simulink model "Streaming_LUT"  (R2024a)
settings: Solver=ode1  StartTime=0.0  StopTime=10  FixedStep=0.001  RelTol=1e-3  EnableMultiTasking=on
PreLoadFcn:
  | a = reshape(1:2800, [4 5 20 7]);
undefined symbols (not defined in the file): xi, yi, ZI
libraries: simulink x2
settings Model: Creator=The MathWorks, Inc.  LastModifiedBy=jjansev
settings SolverCC: AlgebraicLoopSolver=TrustRegion
settings DataIOCC: LimitDataPoints=on  SaveFormat=Array
settings OptimizationCC: ExpressionDepthLimit=2147483647  LifeSpan=inf
settings DebuggingCC: UnderspecifiedInitializationDetection=Classic  MergeDetectMultiDrivingBlocksExec=none  SolverPrmCheckMsg=warning  FcnCallInpInsideContextMsg=warning  UnconnectedInputMsg=warning  UnconnectedOutputMsg=warning  UnconnectedLineMsg=warning  StateNameClashWarn=warning  PregeneratedLibrarySubsystemCodeDiagnostic=none  SFUnexpectedBacktrackingDiag=warning  SFNoUnconditionalDefaultTransitionDiag=warning  SFExecutionAtInitializationDiag=none  ArithmeticOperatorsInVariantConditions=warning
settings HardwareCC: ProdBitPerPointer=32  ProdBitPerSizeT=32  ProdBitPerPtrDiffT=32  ProdLargestAtomicFloat=None  ProdIntDivRoundTo=Undefined  ProdEndianess=Unspecified  ProdWordSize=32  ProdHWDeviceType=32-bit Generic
settings ModelReferenceCC: EnableRefExpFcnMdlSchedulingChecks=on  PropagateSignalLabelsOutOfModel=off
settings SFSimCC: SimUseLocalCustomCode=off  CustomCodeUndefinedFunction=UseInterfaceOnly
settings RTWCC: RTWUseLocalCustomCode=off  GPUComputeCapability=3.5
settings CodeAppCC: StateflowObjectComments=on
settings GRTTargetCC: TargetLangStandard=C89/C90 (ANSI)  CombineOutputUpdateFcns=off  GRTInterface=on
settings ConfigComp: CovMetricSettings=dw  CovSaveCumulativeToWorkspaceVar=on  CovSaveSingleToWorkspaceVar=on  CovExternalEMLEnable=off

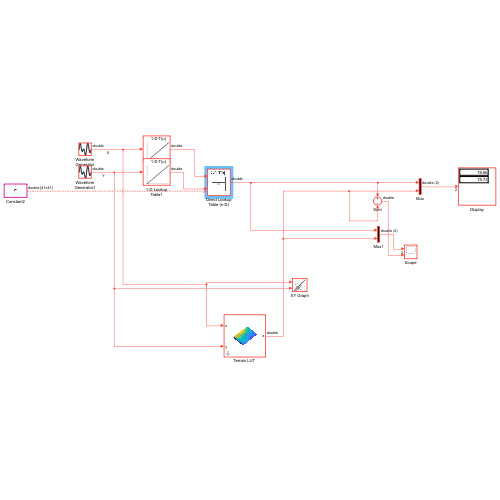
[thumbnail: Simulink's stored preview of the top-level diagram]
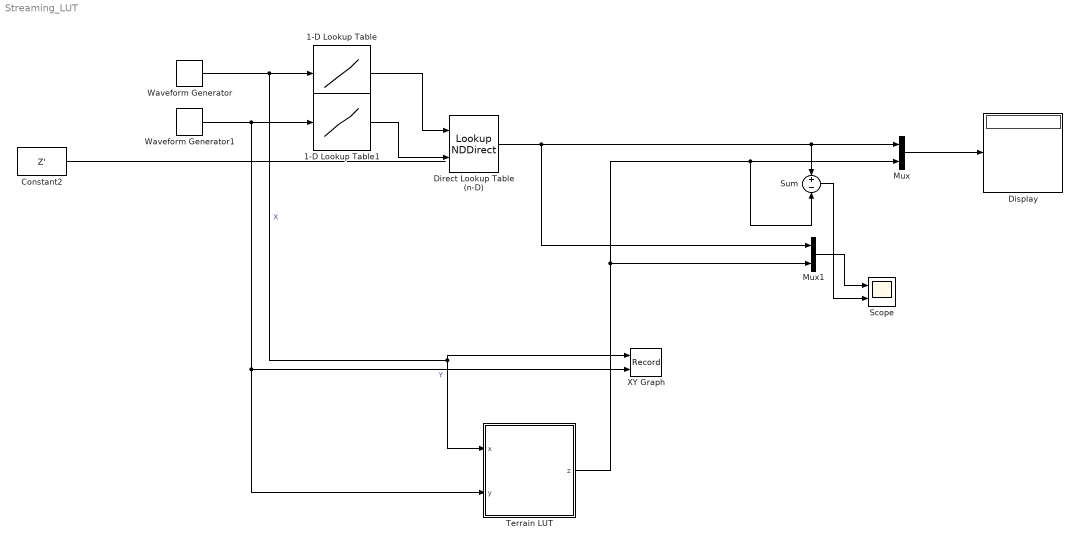
== system Streaming_LUT ==
  1-D Lookup Table : Lookup_n-D  NumberOfTableDimensions=1  BreakpointsForDimension1=[-10 10]  Table=[1 41]  InternalRulePriority=Speed  RndMeth=Simplest
  1-D Lookup Table1 : Lookup_n-D  NumberOfTableDimensions=1  BreakpointsForDimension1=[-10 10]  Table=[1 41]  InternalRulePriority=Speed  RndMeth=Simplest
  Constant2 : Constant  Value=Z'
  Direct Lookup Table (n-D) : LookupNDDirect  Table=Z'
  Display : Display
  Mux : Mux  Inputs=2
  Mux1 : Mux  Inputs=2
  Scope : Scope  NumInputPorts=2
  Sum : Sum  Inputs=+-
  "Terrain LUT " : Subsystem  AncestorBlock=|  mask{stlFileName='MRC_t.stl', resolution=5, color=[0.5 0.5 0.6], x_query=0, y_query=0, Int_method=Linear}
      | PC_GS_SSMB/TerrainFromSTL 
      | (Visuzalize GridSurface)
      mask prompts: stlFileName "STL Filename"; resolution "Resolution of the Grid surface [m]"; color "Color of the Grid-surface"; x_query "Position on x-axis to be polled for z-height (Frame F1)"; y_query "Position on y-axis to be polled for z-height (Frame F1)"; Int_method "Interpolation method Used of the Surface"
      mask init:
      | % Use set_param to set the parameter
      | [imageMatrix, xi, yi, ZI, Res_orig, z_query] = GenerateTerrainFromSTL(stlFileName, resolution, x_query, y_query, Int_method);
      mask Display: image(imageMatrix);
  Waveform Generator : simulink/Sources/Waveform Generator  OutMin=[]  OutMax=[]  OutDataTypeStr=double  SelectedSignal=1  Signals=sin(10.0,5,0)  BlockNames=MultiportSwitch_dd9a2ba7f6ab439  SampleTime=0.001
  Waveform Generator1 : simulink/Sources/Waveform Generator  OutMin=[]  OutMax=[]  OutDataTypeStr=double  SelectedSignal=2  Signals=sin(40,5,0)#sin(10.0,3,pi/2)  BlockNames=MultiportSwitch_ab584ca8b97949d#MultiportSwitch_da390b7282c442c  SampleTime=0.001
  XY Graph : Record  FileSettingsInternal="{\"entries\":[{\"content\":{\"excelSettings\":{\"content\":{},\"type\":\"Streamout.ExcelSettings\"}},\"type\":\"Streamout.FileSettingStorage\",\"uuid\":\"\"}],\"packageUris\":[\"http:\\/\\/schema.mathworks.com\\/mf0\\/streamout_blocks\\/R2020a\"],\"version\":\"1.0\"}"  Layout=[1 1]  SignalsInternal="{\"entries\":[{\"content\":{\"signals\":[{\"content\":{\"blockPath\":[],\"dimensions\":[1],\"domain\":\"\",\"lineColor\":\"#a2142f\",\"plots\":[ 1 ],\"port\":1,\"sid\":[\"\"],\"signalID\":1,\"signalName\":\"X\"},\"type\":\"RecordBlkView.Signal\",\"uuid\":\"\"},{\"content\":{\"blockPath\":[],\"dimensions\":[1],\"domain\":\"\",\"lineColor\":\"#139fff\",\"plots\":[ 1 ],\"port\":2,\"sid\":[\"\"],\"signalID\":2,\"signalName\":\"Y\"},\"type\":\"RecordBlkView.Signal\",\"uuid\":\"\"}]},\"type\":\"RecordBlkView.InputSignals\",\"uuid\":\"\"}],\"packageUris\":[\"http:\\/\\/schema.mathworks.com\\/mf0\\/streamout_blocks\\/R2020a\"],\"version\":\"1.0\"}"  VisualizationBindings="{\"xyplotplugin\":{\"info\":[{\"series\":[{\"bindingParametersList\":[{\"parameter\":\"X-Axis\",\"signalID\":1,\"signalName\":\"X\"},{\"parameter\":\"Y-Axis\",\"signalID\":2,\"signalName\":\"Y\"}],\"seriesID\":0}],\"subplotID\":1}]}}"  CompatibilityTag=XY
  wires:
  Waveform Generator1/1 -> 1-D Lookup Table1/1, "Terrain LUT "/2(y), XY Graph/2  "Y"
  Constant2/1 -> ?
  Direct Lookup Table (n-D)/1 -> Mux1/1, Sum/1, Mux/1
  "Terrain LUT "/1(z) -> Mux1/2, Sum/2, Mux/2
  Mux/1 -> Display/1
  Waveform Generator/1 -> 1-D Lookup Table/1, "Terrain LUT "/1(x), XY Graph/1  "X"
  1-D Lookup Table/1 -> Direct Lookup Table (n-D)/1
  1-D Lookup Table1/1 -> Direct Lookup Table (n-D)/2
  Mux1/1 -> Scope/1
  Sum/1 -> Scope/2

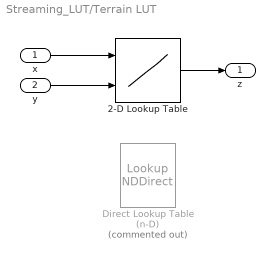
== system Streaming_LUT/Terrain LUT  ==
  x : Inport
  y : Inport  Port=2
  2-D Lookup Table : Lookup_n-D  BreakpointsForDimension1=xi  BreakpointsForDimension2=yi  Table=ZI'  InternalRulePriority=Speed  RndMeth=Simplest
      settings: InputPortMap=u0,u1
  Direct Lookup Table (n-D) : LookupNDDirect  Commented=on  Table=[ZI]
  z : Outport
  wires:
  x/1 -> 2-D Lookup Table/1
  y/1 -> 2-D Lookup Table/2
  2-D Lookup Table/1 -> z/1
